simulink model "PID_diagrama_de_blocos"  (R2020a)
settings: Solver=VariableStepAuto  StartTime=0.0  StopTime=20  RelTol=1e-3
settings Model: Creator=crist  LastModifiedBy=crist
settings SolverCC: ZeroCrossAlgorithm=Adaptive

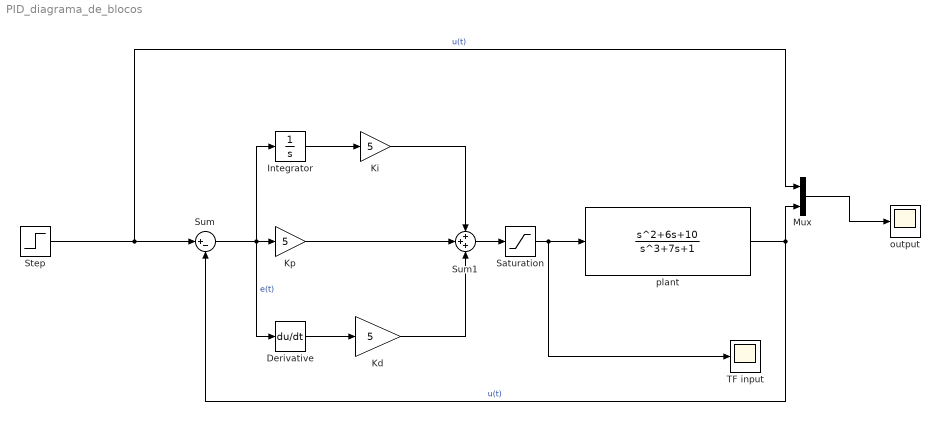
== system PID_diagrama_de_blocos ==
  Derivative : Derivative
  Integrator : Integrator
  Kd : Gain  Gain=5
  Ki : Gain  Gain=5
  Kp : Gain  Gain=5
  Mux : Mux  Inputs=2
  Saturation : Saturate  UpperLimit=2  LowerLimit=-2
  Step : Step  SampleTime=0
  Sum : Sum  Inputs=|+-
  Sum1 : Sum  Inputs=+++
  TF input : Scope
  output : Scope
  plant : TransferFcn  Numerator=[1 6 10]  Denominator=[1 0 7 1]
  wires:
  Sum/1 -> Integrator/1, Derivative/1, Kp/1  "e(t)"
  plant/1 -> Mux/2, Sum/2  "u(t)"
  Step/1 -> Mux/1, Sum/1  "u(t)"
  Mux/1 -> output/1
  Ki/1 -> Sum1/1
  Kd/1 -> Sum1/3
  Sum1/1 -> Saturation/1
  Kp/1 -> Sum1/2
  Integrator/1 -> Ki/1
  Derivative/1 -> Kd/1
  Saturation/1 -> TF input/1, plant/1
